simulink model "FluxModel2015a_verify_Q_zhixin"  (R2020b)
settings: Solver=VariableStepAuto  StartTime=0.0  StopTime=0.3  FixedStep=Ts  RelTol=1e-3  EnableMultiTasking=on
model workspace (MAT data in the model file):
  MOVE : Simulink.Parameter (value not decoded)
  STOP : Simulink.Parameter (value not decoded)
  thres : Simulink.Parameter (value not decoded)
values from neighbouring files (symbols this model uses):
  AngleEncoderEn = 1    [parameters.m]
  AngleSpdClosedLoopEnable = 0.0    (= 0)    [parameters.m]
  CurrentLoopMax = Q14*1.2    (= 19660.8)    [parameters.m]
  EstOutMax_Speed_Q = Q14*1.2    (= 19660.8)    [parameters.m]
  Factor1 = Q15*Ts*Rb/Lq_realvalue    [parameters.m]
  Factor2 = Q15*Ts*Rs_realvalue/Lq_realvalue    (= 16990.2962963)    [parameters.m]
  fieldweaken_Max = 0    [parameters.m]
  fieldweaken_Min = -0.5*Q14    (= -8192)    [parameters.m]
  FieldWeakenEn = 0    [parameters.m]
  fluxF = Lam_realvalue/fluxB    [parameters.m]
  fluxF_Q14 = Q14*fluxF    [parameters.m]
  Friction = 0.003    [parameters.m]
  Ib = sqrt(2)*In    [parameters.m]
  Id_Ki = Q14*CurrentLoopBandwidth*Rs    [parameters.m]
  Id_Kp = Q14*CurrentLoopBandwidth*Ld    [parameters.m]
  IFCurrDecreased = 1    [parameters.m]
  IFCurrStart = 8    [parameters.m]
  IFCurrTarget = 5    [parameters.m]
  IFIdref = 0    [parameters.m]
  initial_degree = 0    [parameters.m]
  Iq_Ki = Q14*CurrentLoopBandwidth*Rs    [parameters.m]
  Iq_Kp = Q14*CurrentLoopBandwidth*Lq    [parameters.m]
  J_realvalue = 2.47e-4    (= 0.000247)    [parameters.m]
  KI_fieldweaken = 0.1*Q14    (= 1638.4)    [parameters.m]
  KP_fieldweaken = 1.0*Q14    (= 16384)    [parameters.m]
  LamObserverGain_Q = Q15*LamObserverGain    (= 13106.8)    [parameters.m]
  Ld = Ld_realvalue/Lb    [parameters.m]
  Ld_Q14 = Q14*Ld_realvalue/Lb    [parameters.m]
  Ld_realvalue = 2.7e-3    (= 0.0027)    [parameters.m]
  LowPassFilterBandWidth_Emf_Q = Q14*LowPassFilterBandWidth_Emf    (= 1445.64705882)    [parameters.m]
  LowPassFilterCoeff_Emf = Q15*(1/(1+LowPassFilterBandWidth_Emf*TsPu))    (= 31292.3812732)    [parameters.m]
  LowPassFilterCoeff_Spd = Q15*(1/(1+LowPassFilterBandWidth_Speed*SpeedloopTs/tb))    (= 20123.2126159)    [parameters.m]
  Lq = Lq_realvalue/Lb    [parameters.m]
  Lq_Q14 = Q14*Lq_realvalue/Lb    [parameters.m]
  Lq_realvalue = 2.7e-3    (= 0.0027)    [parameters.m]
  MOVE = 1    [parameters.m]
  Np = 1    [parameters.m]
  Omega0_Q = Q14*Omega0    (= 6553.6)    [parameters.m]
  OverModulationEn = 0    [parameters.m]
  PLL_KI = Q14*PLL_Bandwidth*PLL_Bandwidth    (= 56.6920415225)    [parameters.m]
  PLL_KP = Q14*2*PLL_Bandwidth    (= 1927.52941176)    [parameters.m]
  PLL_OUTMax_W = Q14*1.2    (= 19660.8)    [parameters.m]
  PWM_Period = 1000    [parameters.m]
  Q14 = 16384    [parameters.m]
  Q15 = 32767    [parameters.m]
  Q16 = 65535    [parameters.m]
  Rs = Rs_realvalue/Rb    [parameters.m]
  Rs_Q14 = Q14*Rs_realvalue/Rb    [parameters.m]
  Rs_realvalue = 28    [parameters.m]
  SecondOverMod = 0    [parameters.m]
  SMO_Gain = Q14*0.85    (= 13926.4)    [parameters.m]
  SMO_I_ERROR = Q14*0.05    (= 819.2)    [parameters.m]
  SpdClosedLoopEnable = 0.0    (= 0)    [parameters.m]
  Speed_Ki = Q14*SpeedLoopBandwidth    (= 481.882352941)    [parameters.m]
  Speed_Kp = Q14*SpeedLoopBandwidth*JPu/fluxF    [parameters.m]
  SpeedIncreased = 0.1*Wb    (= 1068.14150222)    [parameters.m]
  SpeedloopTs = 1/SpeedloopFrequency    (= 0.001)    [parameters.m]
  Speedn = 60*fn/Np    (= 102000)    [parameters.m]
  SpeedOutmax = 1.2*Q14    (= 19660.8)    [parameters.m]
  SpeedSwitch = 0.6*Wb    (= 6408.84901332)    [parameters.m]
  SpeedTarget = 0.8*Wb    (= 8545.13201776)    [parameters.m]
  STOP = 0    [parameters.m]
  SVCM_GAIN_Q = Q15*SVCM_GAIN    (= 26213.6)    [parameters.m]
  tb = 1/Wb    (= 9.36205547599e-05)    [parameters.m]
  Tf = 0    [parameters.m]
  thres = 0.1    [parameters.m]
  Tn = 0.012    [parameters.m]
  Ts = 1/SwitchFrequency    (= 5e-05)    [parameters.m]
  TsPu = Ts/tb    (= 0.53407075111)    [parameters.m]
  Vb = Vdc/sqrt(3)    [parameters.m]
  Vdc = sqrt(2)*Un    [parameters.m]
  Wb = 2*pi*fn    (= 10681.4150222)    [parameters.m]
  ZeroSeqInjectEn = 0.0    (= 0)    [parameters.m]
undefined symbols (not defined in the file or in its folder): DiscIntNeverNeededParam, EstOutMax_Theta, magnitude, sigbuilder_block
libraries: simulink x9, powerlib x5, mcbutilslib x1
(part 2 of 3)

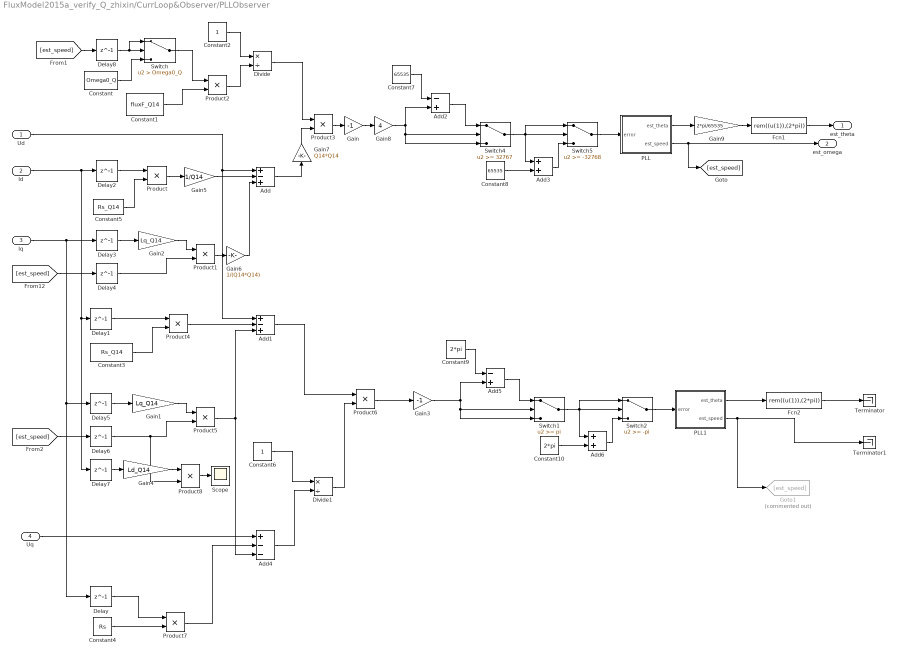
== system FluxModel2015a_verify_Q_zhixin/CurrLoop&Observer/PLLObserver ==
  Ud : Inport
  Id : Inport  Port=2
  Iq : Inport  Port=3
  Uq : Inport  Port=4
  Add : Sum  Inputs=+-+
  Add1 : Sum  Inputs=+-+
  Add2 : Sum  Inputs=-+
  Add3 : Sum
  Add4 : Sum  Inputs=+--
  Add5 : Sum  Inputs=-+
  Add6 : Sum
  Constant : Constant  Value=Omega0_Q
  Constant1 : Constant  Value=fluxF_Q14
  Constant10 : Constant  Value=2*pi
  Constant2 : Constant
  Constant3 : Constant  Value=Rs_Q14
  Constant4 : Constant  Value=Rs
  Constant5 : Constant  Value=Rs_Q14
  Constant6 : Constant
  Constant7 : Constant  Value=65535
  Constant8 : Constant  Value=65535
  Constant9 : Constant  Value=2*pi
  Delay{,1..8} (9 alike) : Delay  DelayLength=1
  Divide : Product  Inputs=*/
  Divide1 : Product  Inputs=*/
  Fcn1 : Fcn  Expr=rem((u(1)),(2*pi))
  Fcn2 : Fcn  Expr=rem((u(1)),(2*pi))
  Gain : Gain  Gain=-1
  Gain1 : Gain  Gain=Lq_Q14
  Gain2 : Gain  Gain=Lq_Q14
  Gain3 : Gain  Gain=-1
  Gain4 : Gain  Gain=Ld_Q14
  Gain5 : Gain  Gain=1/Q14
  Gain6 : Gain  Gain=1/(Q14*Q14)
  Gain7 : Gain  Gain=Q14*Q14
  Gain8 : Gain  Gain=4
  Gain9 : Gain  Gain=2*pi/65535
  Goto1 : Goto  Commented=on  GotoTag=est_speed
  PLL : Subsystem
  PLL1 : Subsystem
  Product{,1..8} (9 alike) : Product
  Scope : Scope
  Switch : Switch  Criteria=u2 > Threshold  Threshold=Omega0_Q
  Switch1 : Switch  Threshold=pi
  Switch2 : Switch  Threshold=-pi
  Switch4 : Switch  Threshold=32767
  Switch5 : Switch  Threshold=-32768
  Terminator : Terminator
  Terminator1 : Terminator
  est_theta : Outport
  est_omega : Outport  Port=2
  wires:
  Constant5/1 -> Product/2
  [est_speed] -> Delay4/1
  Delay4/1 -> Product1/2
  Gain2/1 -> Product1/1
  Delay3/1 -> Gain2/1
  Product1/1 -> Gain6/1
  Product/1 -> Gain5/1
  Delay2/1 -> Product/1
  Id/1 -> Delay7/1, Delay1/1, Delay2/1
  Add/1 -> Gain7/1
  Delay8/1 -> Switch/1, Switch/2
  Constant/1 -> Switch/3
  Switch/1 -> Product2/1
  Constant1/1 -> Product2/2
  Constant2/1 -> Divide/1
  Product2/1 -> Divide/2
  Divide/1 -> Product3/1
  Switch4/1 -> Switch5/1, Add3/1, Switch5/2
  PLL/2(est_speed) -> est_omega/1, [est_speed]
  Add3/1 -> Switch5/3
  Constant8/1 -> Add3/2
  Constant7/1 -> Add2/1
  Add2/1 -> Switch4/1
  Switch5/1 -> PLL/1(error)
  Product3/1 -> Gain/1
  Gain/1 -> Gain8/1
  PLL/1(est_theta) -> Gain9/1
  Constant3/1 -> Product4/2
  Product4/1 -> Add1/2
  Delay1/1 -> Product4/1
  Ud/1 -> Add1/1, Add/1
  Delay6/1 -> Product8/2, Product5/2
  Gain1/1 -> Product5/1
  Delay5/1 -> Gain1/1
  Iq/1 -> Delay/1, Delay5/1, Delay3/1
  Product5/1 -> Add4/3, Add1/3
  Add1/1 -> Product6/1
  Uq/1 -> Add4/1
  Delay/1 -> Product7/1
  Constant4/1 -> Product7/2
  Product7/1 -> Add4/2
  Constant6/1 -> Divide1/1
  Add4/1 -> Divide1/2
  Divide1/1 -> Product6/2
  Product6/1 -> Gain3/1
  Switch1/1 -> Switch2/1, Add6/1, Switch2/2
  Constant9/1 -> Add5/1
  Constant10/1 -> Add6/2
  Switch2/1 -> PLL1/1(error)
  Add5/1 -> Switch1/1
  Gain3/1 -> Switch1/3, Switch1/2, Add5/2
  Add6/1 -> Switch2/3
  PLL1/1(est_theta) -> Fcn2/1
  Fcn2/1 -> Terminator/1
  PLL1/2(est_speed) -> Terminator1/1, Goto1/1
  Fcn1/1 -> est_theta/1
  Delay7/1 -> Gain4/1
  [est_speed] -> Delay6/1
  Gain4/1 -> Product8/1
  Product8/1 -> Scope/1
  Gain5/1 -> Add/2
  Gain6/1 -> Add/3
  Gain7/1 -> Product3/2
  Gain8/1 -> Switch4/3, Switch4/2, Add2/2
  Gain9/1 -> Fcn1/1
  [est_speed] -> Delay8/1

== system FluxModel2015a_verify_Q_zhixin/CurrLoop&Observer/Park ==
  alpha : Inport
  beta : Inport  Port=2
  theta : Inport  Port=3
  Add : Sum
  Cos : Trigonometry  Operator=cos
  Product{,1..3} (4 alike) : Product
  Sin : Trigonometry
  Subtract1 : Sum  Inputs=+-
  ID : Outport
  IQ : Outport  Port=2
  wires:
  Product2/1 -> Subtract1/1
  beta/1 -> Product2/1, Product/1
  theta/1 -> Cos/1, Sin/1
  Sin/1 -> Product3/2, Product/2
  alpha/1 -> Product3/1, Product1/2
  Cos/1 -> Product1/1, Product2/2
  Subtract1/1 -> IQ/1
  Product1/1 -> Add/2
  Product3/1 -> Subtract1/2
  Product/1 -> Add/1
  Add/1 -> ID/1

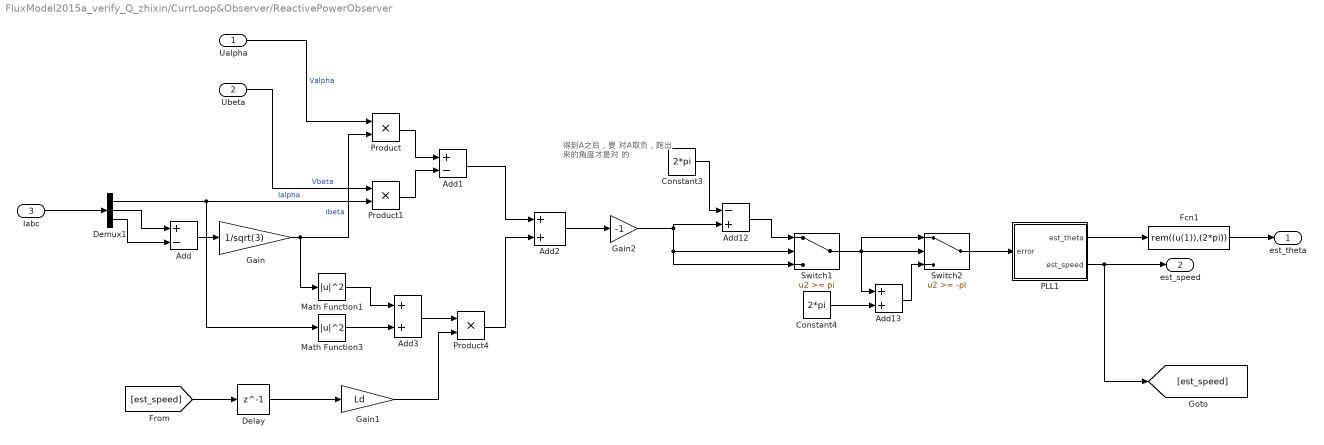
== system FluxModel2015a_verify_Q_zhixin/CurrLoop&Observer/ReactivePowerObserver ==
  note: 得到A之后，要
      | 对A取负，跑出
      | 来的角度才是对
      | 的
  Ualpha : Inport
  Ubeta : Inport  Port=2
  Iabc : Inport  Port=3
  Add : Sum  Inputs=+-
  Add1 : Sum  Inputs=+-
  Add12 : Sum  Inputs=-+
  Add13 : Sum
  Add2 : Sum
  Add3 : Sum
  Constant3 : Constant  Value=2*pi
  Constant4 : Constant  Value=2*pi
  Delay : Delay  DelayLength=1
  Demux1 : Demux  Outputs=3
  Fcn1 : Fcn  Expr=rem((u(1)),(2*pi))
  Gain : Gain  Gain=1/sqrt(3)
  Gain1 : Gain  Gain=Ld
  Gain2 : Gain  Gain=-1
  Math Function1 : Math  Operator=magnitude^2  SaturateOnIntegerOverflow=on
  Math Function3 : Math  Operator=magnitude^2  SaturateOnIntegerOverflow=on
  PLL1 : Subsystem
  Product : Product
  Product1 : Product
  Product4 : Product
  Switch1 : Switch  Threshold=pi
  Switch2 : Switch  Threshold=-pi
  est_theta : Outport
  est_speed : Outport  Port=2
  wires:
  Demux1/1 -> Product1/2, Math Function3/1  "Ialpha"
  Product1/1 -> Add1/2
  Math Function1/1 -> Add3/1
  Demux1/2 -> Add/1
  Gain/1 -> Product/2, Math Function1/1  "Ibeta"
  Add1/1 -> Add2/1
  Ubeta/1 -> Product1/1  "Vbeta"
  Ualpha/1 -> Product/1  "Valpha"
  Product/1 -> Add1/1
  Add/1 -> Gain/1
  Demux1/3 -> Add/2
  Product4/1 -> Add2/2
  Add3/1 -> Product4/1
  Gain1/1 -> Product4/2
  Iabc/1 -> Demux1/1
  Constant4/1 -> Add13/2
  Switch2/1 -> PLL1/1(error)
  Switch1/1 -> Switch2/1, Add13/1, Switch2/2
  PLL1/1(est_theta) -> Fcn1/1
  Constant3/1 -> Add12/1
  Add12/1 -> Switch1/1
  PLL1/2(est_speed) -> [est_speed], est_speed/1
  Add13/1 -> Switch2/3
  Math Function3/1 -> Add3/2
  Fcn1/1 -> est_theta/1
  [est_speed] -> Delay/1
  Delay/1 -> Gain1/1
  Add2/1 -> Gain2/1
  Gain2/1 -> Switch1/3, Switch1/2, Add12/2

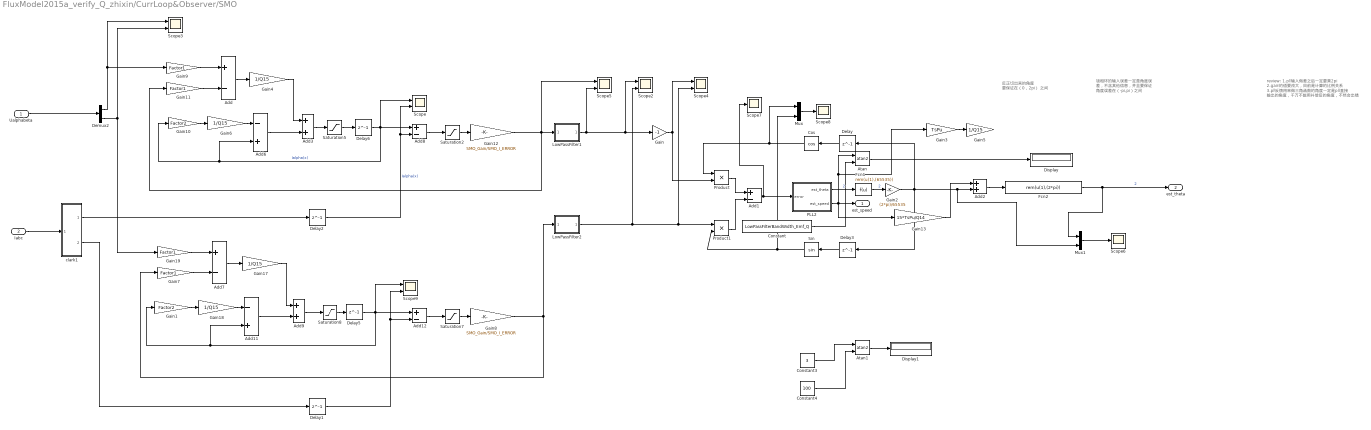
== system FluxModel2015a_verify_Q_zhixin/CurrLoop&Observer/SMO ==
  note: 反正切出来的角度
      | 要保证在（0，2pi）
      | 之间
  note: 锁相环的输入误差一定是角度误
      | 差，不含其他信息，并且要保证
      | 角度误差在（-pi,pi）之间
  note: review:
      | 1.pll输入做差之后一定要乘2pi
      | 2.gain的值要改大，目前是计算的比例关系
      | 3.pll反馈用来做三角函数的角度一定是pll直接
      | 输出的角度，千万不能用补偿后的角度，不然会出错
  Ualphabeta : Inport
  Iabc : Inport  Port=2
  Add{,1,7..8,12} (5 alike) : Sum  Inputs=+-
  Add11 : Sum  Inputs=-+
  Add2 : Sum
  Add3 : Sum
  Add6 : Sum  Inputs=-+
  Add9 : Sum
  Atan : Trigonometry  Operator=atan2
  Atan1 : Trigonometry  Operator=atan2
  Constant : Constant  Value=LowPassFilterBandWidth_Emf_Q
  Constant3 : Constant  Value=3
  Constant4 : Constant  Value=100
  Cos : Trigonometry  Operator=cos
  Delay{,1..3,5..6} (6 alike) : Delay  DelayLength=1
  Demux2 : Demux  Outputs=2
  Display : Display
  Display1 : Display
  Fcn1 : Fcn  Expr=rem(u(1),(65535))
  Fcn2 : Fcn  Expr=rem(u(1),(2*pi))
  Gain : Gain  Gain=-1
  Gain1 : Gain  Gain=Factor2
  Gain10 : Gain  Gain=Factor2
  Gain{7,9,11,19} (4 alike) : Gain  Gain=Factor1
  Gain12 : Gain  Gain=SMO_Gain/SMO_I_ERROR
  Gain13 : Gain  Gain=15*TsPu/Q14
  Gain{4..6,17..18} (5 alike) : Gain  Gain=1/Q15
  Gain2 : Gain  Gain=(2*pi)/65535
  Gain3 : Gain  Gain=TsPu
  Gain8 : Gain  Gain=SMO_Gain/SMO_I_ERROR
  LowPassFilter1 : Subsystem
  LowPassFilter2 : Subsystem
  Mux : Mux  Inputs=2
  Mux1 : Mux  Inputs=2
  PLL2 : Subsystem
  Product : Product
  Product1 : Product
  Saturation2 : Saturate  UpperLimit=SMO_I_ERROR  LowerLimit=-SMO_I_ERROR
  Saturation5 : Saturate  UpperLimit=16384  LowerLimit=-16384
  Saturation7 : Saturate  UpperLimit=SMO_I_ERROR  LowerLimit=-SMO_I_ERROR
  Saturation8 : Saturate  UpperLimit=16384  LowerLimit=-16384
  Scope{,2..5,9} (6 alike) : Scope  NumInputPorts=2
  Scope6 : Scope
  Scope7 : Scope
  Scope8 : Scope
  Sin : Trigonometry
  clark1 : Subsystem
  est_speed : Outport
  est_theta : Outport  Port=2
  wires:
  Demux2/1 -> Scope3/1, Gain9/1
  Gain9/1 -> Add/1
  Saturation2/1 -> Gain12/1
  Gain11/1 -> Add/2
  Add8/1 -> Saturation2/1
  Delay6/1 -> Scope/1, Add8/1, Add6/2, Gain10/1  "Ialpha(x)"
  Delay/1 -> Cos/1
  Cos/1 -> Mux/1, Product/1
  Delay3/1 -> Sin/1
  Sin/1 -> Mux/2, Product1/2
  Product/1 -> Add1/1
  Product1/1 -> Add1/2
  PLL2/2(est_speed) -> Gain13/1, Gain3/1, Atan/1, est_speed/1
  Add1/1 -> PLL2/1(error), Scope7/1
  PLL2/1(est_theta) -> Fcn1/1  "2"
  Constant/1 -> Atan/2
  Fcn2/1 -> Mux1/1, est_theta/1  "2"
  Add2/1 -> Fcn2/1
  Constant3/1 -> Atan1/1
  Constant4/1 -> Atan1/2
  Atan1/1 -> Display1/1
  LowPassFilter1/1(Output) -> Scope5/2, Scope2/1, Gain/1
  Add/1 -> Gain4/1
  Gain4/1 -> Add3/1
  Ualphabeta/1 -> Demux2/1
  Iabc/1 -> clark1/1(Iabc)
  Delay2/1 -> Scope/2, Add8/2  "Ialpha(x)"
  Gain/1 -> Product/2, Scope4/1
  LowPassFilter2/1(Output) -> Scope2/2, Product1/1, Scope4/2
  Mux/1 -> Scope8/1
  Atan/1 -> Display/1
  clark1/1(Ialpha) -> Delay2/1
  Gain12/1 -> Scope5/1, LowPassFilter1/1(Input), Gain11/1
  Add6/1 -> Add3/2
  Gain10/1 -> Gain6/1
  Gain6/1 -> Add6/1
  Add11/1 -> Add9/2
  Gain1/1 -> Gain18/1
  Gain18/1 -> Add11/1
  Gain7/1 -> Add7/2
  clark1/2(Ibeta) -> Delay1/1
  Gain8/1 -> LowPassFilter2/1(Input), Gain7/1
  Saturation7/1 -> Gain8/1
  Add7/1 -> Gain17/1
  Gain17/1 -> Add9/1
  Delay5/1 -> Scope9/1, Add12/1, Add11/2, Gain1/1
  Gain19/1 -> Add7/1
  Demux2/2 -> Gain19/1, Scope3/2
  Add12/1 -> Saturation7/1
  Delay1/1 -> Scope9/2, Add12/2
  Add3/1 -> Saturation5/1
  Saturation5/1 -> Delay6/1
  Add9/1 -> Saturation8/1
  Saturation8/1 -> Delay5/1
  Fcn1/1 -> Gain2/1  "2"
  Mux1/1 -> Scope6/1
  Gain3/1 -> Gain5/1
  Gain2/1 -> Mux1/2, Add2/2, Delay3/1, Delay/1
  Gain13/1 -> Add2/1

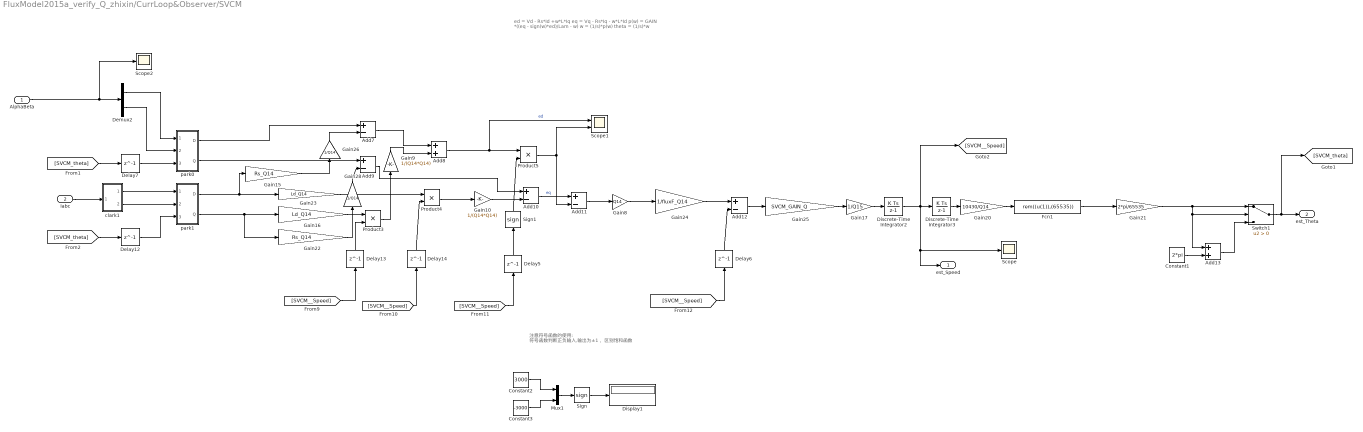
== system FluxModel2015a_verify_Q_zhixin/CurrLoop&Observer/SVCM ==
  note: 注意符号函数的使用:
      | 符号函数判断正负输入,输出为±1，
      | 区别饱和函数
  note: ed = Vd - Rs*Id +w*L*Iq
      | eq = Vq - Rs*Iq - w*L*Id
      | p(w) = GAIN *((eq - sign(w)*ed)/Lam - w)
      | w = (1/s)*p(w)
      | theta = (1/s)*w
  AlphaBeta : Inport
  Iabc : Inport  Port=2
  Add{7,9..12} (5 alike) : Sum  Inputs=+-
  Add13 : Sum
  Add8 : Sum
  Constant1 : Constant  Value=2*pi
  Constant2 : Constant  Value=3000
  Constant3 : Constant  Value=-3000
  Delay{5..7,12..14} (6 alike) : Delay  DelayLength=1
  Demux2 : Demux  Outputs=2
  Discrete-Time Integrator2 : DiscreteIntegrator  gainval=1.0/tb  SampleTime=-1  LimitOutput=on  UpperSaturationLimit=EstOutMax_Speed_Q  LowerSaturationLimit=-EstOutMax_Speed_Q  ICPrevOutput=DiscIntNeverNeededParam  ICPrevScaledInput=DiscIntNeverNeededParam
  Discrete-Time Integrator3 : DiscreteIntegrator  gainval=1.0/tb  SampleTime=-1  UpperSaturationLimit=EstOutMax_Theta  LowerSaturationLimit=-EstOutMax_Theta  ICPrevOutput=DiscIntNeverNeededParam  ICPrevScaledInput=DiscIntNeverNeededParam
  Display1 : Display
      settings: Decimation=2
  Fcn1 : Fcn  Expr=rem((u(1)),(65535))
  Gain10 : Gain  Gain=1/(Q14*Q14)
  Gain15 : Gain  Gain=Rs_Q14
  Gain16 : Gain  Gain=Ld_Q14
  Gain17 : Gain  Gain=1/Q15
  Gain20 : Gain  Gain=10430/Q14
  Gain21 : Gain  Gain=2*pi/65535
  Gain22 : Gain  Gain=Rs_Q14
  Gain23 : Gain  Gain=Ld_Q14
  Gain24 : Gain  Gain=1/fluxF_Q14
  Gain25 : Gain  Gain=SVCM_GAIN_Q
  Gain26 : Gain  Gain=1/Q14
  Gain28 : Gain  Gain=1/Q14
  Gain8 : Gain  Gain=Q14
  Gain9 : Gain  Gain=1/(Q14*Q14)
  Mux1 : Mux  Inputs=2
  Product3 : Product
  Product4 : Product
  Product5 : Product
  Scope : Scope
  Scope1 : Scope  NumInputPorts=2
  Scope2 : Scope
  Sign : Signum
  Sign1 : Signum
  Switch1 : Switch  Criteria=u2 > Threshold
  clark1 : Subsystem
  park0 : Subsystem
  park1 : Subsystem
  est_Speed : Outport
  est_Theta : Outport  Port=2
  wires:
  Gain25/1 -> Gain17/1
  Discrete-Time Integrator3/1 -> Gain20/1
  Product3/1 -> Gain9/1
  Gain26/1 -> Add7/2
  Gain28/1 -> Add9/2
  Switch1/1 -> est_Theta/1, [SVCM_theta]
  Delay14/1 -> Product4/2
  Add13/1 -> Switch1/3
  Demux2/1 -> park0/1(alpha)
  Demux2/2 -> park0/2(beta)
  Delay7/1 -> park0/3(theta)
  Delay12/1 -> park1/3(theta)
  [SVCM_theta] -> Delay7/1
  Gain15/1 -> Gain26/1
  Add11/1 -> Gain8/1
  clark1/2(Ibeta) -> park1/2(beta)
  [SVCM__Speed] -> Delay6/1
  clark1/1(Ialpha) -> park1/1(alpha)
  Product4/1 -> Gain10/1
  Gain22/1 -> Gain28/1
  Add12/1 -> Gain25/1
  Add7/1 -> Add8/1
  Add10/1 -> Add11/1  "eq"
  Add8/1 -> Scope1/1, Product5/1  "ed"
  Constant1/1 -> Add13/2
  [SVCM_theta] -> Delay12/1
  Gain24/1 -> Add12/1
  Gain16/1 -> Product3/1
  Delay6/1 -> Add12/2
  Add9/1 -> Add10/1
  Gain23/1 -> Product4/1
  Delay13/1 -> Product3/2
  Iabc/1 -> clark1/1(Iabc)
  Fcn1/1 -> Gain21/1
  Gain20/1 -> Fcn1/1
  Gain21/1 -> Switch1/1, Add13/1, Switch1/2
  Discrete-Time Integrator2/1 -> Scope/1, est_Speed/1, [SVCM__Speed], Discrete-Time Integrator3/1
  Gain9/1 -> Add8/2
  Gain10/1 -> Add10/2
  [SVCM__Speed] -> Delay13/1
  [SVCM__Speed] -> Delay14/1
  [SVCM__Speed] -> Delay5/1
  Product5/1 -> Add11/2, Scope1/2
  Sign1/1 -> Product5/2
  Delay5/1 -> Sign1/1
  Gain8/1 -> Gain24/1
  Gain17/1 -> Discrete-Time Integrator2/1
  Sign/1 -> Display1/1
  Constant2/1 -> Mux1/1
  Constant3/1 -> Mux1/2
  Mux1/1 -> Sign/1
  AlphaBeta/1 -> Scope2/1, Demux2/1
  park0/1(D) -> Add7/1
  park0/2(Q) -> Add9/1
  park1/1(D) -> Gain23/1, Gain15/1
  park1/2(Q) -> Gain22/1, Gain16/1

== system FluxModel2015a_verify_Q_zhixin/CurrLoop&Observer/Subsystem ==
  err : Inport
  Constant14 : Constant  Value=2*pi
  Constant15 : Constant  Value=pi
  Divide4 : Product  Inputs=*/
  Gain5 : Gain  Gain=180
  Math Function6 : Math  Operator=rem  SaturateOnIntegerOverflow=on
  err_Theta : Outport
  err_Rad : Outport  Port=2
  wires:
  Divide4/1 -> Gain5/1
  Constant15/1 -> Divide4/2
  err/1 -> Math Function6/1
  Math Function6/1 -> err_Rad/1, Divide4/1  "err_Theta"
  Constant14/1 -> Math Function6/2
  Gain5/1 -> err_Theta/1

== system FluxModel2015a_verify_Q_zhixin/CurrLoop&Observer/Subsystem1 ==
  err : Inport
  Constant14 : Constant  Value=2*pi
  Constant15 : Constant  Value=pi
  Divide4 : Product  Inputs=*/
  Gain5 : Gain  Gain=180
  Math Function6 : Math  Operator=rem  SaturateOnIntegerOverflow=on
  err_Theta : Outport
  err_Rad : Outport  Port=2
  wires:
  Gain5/1 -> err_Theta/1
  Constant14/1 -> Math Function6/2
  Math Function6/1 -> Divide4/1, err_Rad/1  "err_Theta"
  err/1 -> Math Function6/1
  Constant15/1 -> Divide4/2
  Divide4/1 -> Gain5/1

== system FluxModel2015a_verify_Q_zhixin/CurrLoop&Observer/Subsystem2 ==
  err : Inport
  Constant14 : Constant  Value=2*pi
  Constant15 : Constant  Value=pi
  Divide4 : Product  Inputs=*/
  Gain5 : Gain  Gain=180
  Math Function6 : Math  Operator=rem  SaturateOnIntegerOverflow=on
  err_Theta : Outport
  err_Rad : Outport  Port=2
  wires:
  Divide4/1 -> Gain5/1
  Constant15/1 -> Divide4/2
  err/1 -> Math Function6/1
  Math Function6/1 -> err_Rad/1, Divide4/1  "err_Theta"
  Constant14/1 -> Math Function6/2
  Gain5/1 -> err_Theta/1

== system FluxModel2015a_verify_Q_zhixin/CurrLoop&Observer/Subsystem3 ==
  err : Inport
  Constant14 : Constant  Value=2*pi
  Constant15 : Constant  Value=pi
  Divide4 : Product  Inputs=*/
  Gain5 : Gain  Gain=180
  Math Function6 : Math  Operator=rem  SaturateOnIntegerOverflow=on
  err_Theta : Outport
  err_Rad : Outport  Port=2
  wires:
  Gain5/1 -> err_Theta/1
  Constant14/1 -> Math Function6/2
  Math Function6/1 -> Divide4/1, err_Rad/1  "err_Theta"
  err/1 -> Math Function6/1
  Constant15/1 -> Divide4/2
  Divide4/1 -> Gain5/1

== system FluxModel2015a_verify_Q_zhixin/CurrLoop&Observer/Subsystem4 ==
  err : Inport
  Constant14 : Constant  Value=2*pi
  Constant15 : Constant  Value=pi
  Divide4 : Product  Inputs=*/
  Gain5 : Gain  Gain=180
  Math Function6 : Math  Operator=rem  SaturateOnIntegerOverflow=on
  err_Theta : Outport
  err_Rad : Outport  Port=2
  wires:
  Divide4/1 -> Gain5/1
  Constant15/1 -> Divide4/2
  err/1 -> Math Function6/1
  Math Function6/1 -> err_Rad/1, Divide4/1  "err_Theta"
  Constant14/1 -> Math Function6/2
  Gain5/1 -> err_Theta/1

== system FluxModel2015a_verify_Q_zhixin/CurrLoop&Observer/Subsystem5 ==
  err : Inport
  Gain1 : Gain  Gain=Wb
  Gain2 : Gain  Gain=1/(2*pi)
  Gain3 : Gain  Gain=60/Np
  err_Spd : Outport
  err_Fhz : Outport  Port=2
  wires:
  err/1 -> Gain1/1
  Gain2/1 -> err_Fhz/1, Gain3/1
  Gain1/1 -> Gain2/1
  Gain3/1 -> err_Spd/1

== system FluxModel2015a_verify_Q_zhixin/CurrLoop&Observer/Subsystem6 ==
  err : Inport
  Gain1 : Gain  Gain=Wb
  Gain2 : Gain  Gain=1/(2*pi)
  Gain3 : Gain  Gain=60/Np
  err_Spd : Outport
  err_Fhz : Outport  Port=2
  wires:
  Gain3/1 -> err_Spd/1
  Gain1/1 -> Gain2/1
  Gain2/1 -> Gain3/1, err_Fhz/1
  err/1 -> Gain1/1

== system FluxModel2015a_verify_Q_zhixin/CurrLoop&Observer/Subsystem7 ==
  err : Inport
  Gain1 : Gain  Gain=Wb
  Gain2 : Gain  Gain=1/(2*pi)
  Gain3 : Gain  Gain=60/Np
  err_Spd : Outport
  err_Fhz : Outport  Port=2
  wires:
  err/1 -> Gain1/1
  Gain2/1 -> err_Fhz/1, Gain3/1
  Gain1/1 -> Gain2/1
  Gain3/1 -> err_Spd/1

== system FluxModel2015a_verify_Q_zhixin/CurrLoop&Observer/Subsystem8 ==
  err : Inport
  Gain1 : Gain  Gain=Wb
  Gain2 : Gain  Gain=1/(2*pi)
  Gain3 : Gain  Gain=60/Np
  err_Spd : Outport
  err_Fhz : Outport  Port=2
  wires:
  Gain3/1 -> err_Spd/1
  Gain1/1 -> Gain2/1
  Gain2/1 -> Gain3/1, err_Fhz/1
  err/1 -> Gain1/1

== system FluxModel2015a_verify_Q_zhixin/CurrLoop&Observer/Subsystem9 ==
  err : Inport
  Gain1 : Gain  Gain=Wb
  Gain2 : Gain  Gain=1/(2*pi)
  Gain3 : Gain  Gain=60/Np
  err_Spd : Outport
  err_Fhz : Outport  Port=2
  wires:
  err/1 -> Gain1/1
  Gain2/1 -> err_Fhz/1, Gain3/1
  Gain1/1 -> Gain2/1
  Gain3/1 -> err_Spd/1

== system FluxModel2015a_verify_Q_zhixin/CurrLoop&Observer/ai-park ==
  UD : Inport
  UQ : Inport  Port=2
  The : Inport  Port=3
  Add : Sum
  Cos : Trigonometry  Operator=cos
  Product{,1..3} (4 alike) : Product
  Sin : Trigonometry
  Subtract : Sum  Inputs=+-
  Valpha : Outport
  Vbeta : Outport  Port=2
  wires:
  UQ/1 -> Product3/1, Product1/1
  Product1/1 -> Subtract/2
  Product3/1 -> Add/2
  Cos/1 -> Product3/2, Product/2
  Sin/1 -> Product2/2, Product1/2
  Product/1 -> Subtract/1
  Product2/1 -> Add/1
  The/1 -> Sin/1, Cos/1
  UD/1 -> Product/1, Product2/1
  Subtract/1 -> Valpha/1
  Add/1 -> Vbeta/1

== system FluxModel2015a_verify_Q_zhixin/CurrLoop&Observer/clark ==
  Iabc : Inport
  Add : Sum  Inputs=+-
  Demux2 : Demux  Outputs=3
  Gain : Gain  Gain=18919
  Gain1 : Gain  Gain=1/Q15
  Ialpha : Outport
  Ibeta : Outport  Port=2
  wires:
  Demux2/3 -> Add/2
  Add/1 -> Gain/1
  Demux2/1 -> Ialpha/1
  Demux2/2 -> Add/1
  Gain/1 -> Gain1/1
  Iabc/1 -> Demux2/1
  Gain1/1 -> Ibeta/1

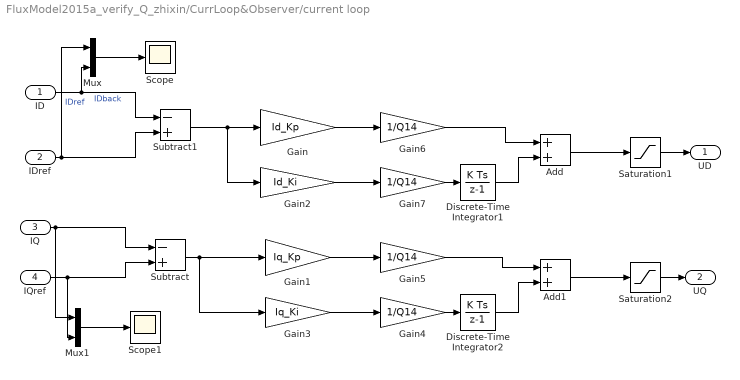
== system FluxModel2015a_verify_Q_zhixin/CurrLoop&Observer/current loop ==
  ID : Inport
  IDref : Inport  Port=2
  IQ : Inport  Port=3
  IQref : Inport  Port=4
  Add : Sum
  Add1 : Sum
  Discrete-Time Integrator1 : DiscreteIntegrator  gainval=1/tb  SampleTime=-1  LimitOutput=on  UpperSaturationLimit=CurrentLoopMax  LowerSaturationLimit=-CurrentLoopMax  ICPrevOutput=DiscIntNeverNeededParam  ICPrevScaledInput=DiscIntNeverNeededParam
  Discrete-Time Integrator2 : DiscreteIntegrator  gainval=1/tb  SampleTime=-1  LimitOutput=on  UpperSaturationLimit=CurrentLoopMax  LowerSaturationLimit=-CurrentLoopMax  ICPrevOutput=DiscIntNeverNeededParam  ICPrevScaledInput=DiscIntNeverNeededParam
  Gain : Gain  Gain=Id_Kp
  Gain1 : Gain  Gain=Iq_Kp
  Gain2 : Gain  Gain=Id_Ki
  Gain3 : Gain  Gain=Iq_Ki
  Gain{4..7} (4 alike) : Gain  Gain=1/Q14
  Mux : Mux  Inputs=2
  Mux1 : Mux  Inputs=2
  Saturation1 : Saturate  UpperLimit=CurrentLoopMax  LowerLimit=-CurrentLoopMax
  Saturation2 : Saturate  UpperLimit=CurrentLoopMax  LowerLimit=-CurrentLoopMax
  Scope : Scope
  Scope1 : Scope
  Subtract : Sum  Inputs=-+
  Subtract1 : Sum  Inputs=-+
  UD : Outport
  UQ : Outport  Port=2
  wires:
  Saturation1/1 -> UD/1
  Subtract1/1 -> Gain/1, Gain2/1
  Saturation2/1 -> UQ/1
  Gain1/1 -> Gain5/1
  Subtract/1 -> Gain3/1, Gain1/1
  Gain/1 -> Gain6/1
  Discrete-Time Integrator1/1 -> Add/2
  Discrete-Time Integrator2/1 -> Add1/2
  IQref/1 -> Mux1/2, Subtract/2
  IDref/1 -> Mux/1, Subtract1/2  "IDref"
  ID/1 -> Mux/2, Subtract1/1  "IDback"
  Mux/1 -> Scope/1
  IQ/1 -> Mux1/1, Subtract/1
  Mux1/1 -> Scope1/1
  Gain3/1 -> Gain4/1
  Add/1 -> Saturation1/1
  Add1/1 -> Saturation2/1
  Gain5/1 -> Add1/1
  Gain4/1 -> Discrete-Time Integrator2/1
  Gain6/1 -> Add/1
  Gain2/1 -> Gain7/1
  Gain7/1 -> Discrete-Time Integrator1/1

== system FluxModel2015a_verify_Q_zhixin/SVPWM/Subsystem ==
  Valpha : Inport
  Vbeta : Inport  Port=2
  Add : Sum  Inputs=+-
  Add1 : Sum  Inputs=+-
  Add2 : Sum  Inputs=+++
  Constant : Constant
  Constant1 : Constant  Value=0
  Gain : Gain  Gain=sqrt(3)
  Gain1 : Gain  Gain=-1
  Gain2 : Gain  Gain=2
  Gain3 : Gain  Gain=4
  Saturation : Saturate  UpperLimit=6  LowerLimit=1
  Switch : Switch  Criteria=u2 > Threshold
  Switch1 : Switch  Criteria=u2 > Threshold
  Switch2 : Switch  Criteria=u2 > Threshold
  N : Outport
  wires:
  Add2/1 -> Saturation/1
  Valpha/1 -> Gain/1
  Gain3/1 -> Add2/2
  Gain2/1 -> Add2/1
  Add1/1 -> Switch1/2
  Gain1/1 -> Add1/1
  Switch1/1 -> Gain3/1
  Switch2/1 -> Add2/3
  Switch/1 -> Gain2/1
  Add/1 -> Switch/2
  Gain/1 -> Gain1/1, Add/1
  Constant1/1 -> Switch/3, Switch1/3, Switch2/3
  Constant/1 -> Switch1/1, Switch2/1, Switch/1
  Vbeta/1 -> Add1/2, Add/2, Switch2/2
  Saturation/1 -> N/1

== system FluxModel2015a_verify_Q_zhixin/SVPWM/Subsystem1 ==
  T : Inport
  In2 : Inport  Port=2
  In3 : Inport  Port=3
  Vdc : Inport  Port=4
  Add : Sum
  Add1 : Sum  Inputs=+-
  Divide : Product  Inputs=**/
  Divide1 : Product  Inputs=**/
  Divide2 : Product  Inputs=**/
  Gain : Gain  Gain=1.732
  Gain1 : Gain  Gain=1.5
  Gain2 : Gain  Gain=0.5
  x : Outport
  Y : Outport  Port=2
  Z : Outport  Port=3
  wires:
  Divide2/1 -> Z/1
  Divide1/1 -> Y/1
  Divide/1 -> x/1
  In3/1 -> Gain1/1
  In2/1 -> Gain/1
  Add1/1 -> Divide2/2
  Add/1 -> Divide1/2
  Gain1/1 -> Add1/2, Add/2
  Gain2/1 -> Add1/1, Add/1
  Gain/1 -> Gain2/1, Divide/2
  Vdc/1 -> Divide/3, Divide1/3, Divide2/3
  T/1 -> Divide2/1, Divide1/1, Divide/1

== system FluxModel2015a_verify_Q_zhixin/SVPWM/Subsystem2 ==
  In1 : Inport
  In2 : Inport  Port=2
  In3 : Inport  Port=3
  In4 : Inport  Port=4
  Gain : Gain  Gain=-1
  Gain1 : Gain  Gain=-1
  Gain2 : Gain  Gain=-1
  Multiport Switch : MultiPortSwitch  Inputs=6
  Multiport Switch1 : MultiPortSwitch  Inputs=6
  T1 : Outport
  T2 : Outport  Port=2
  wires:
  Gain2/1 -> Multiport Switch/7, Multiport Switch1/6
  Gain1/1 -> Multiport Switch1/3, Multiport Switch/5
  In2/1 -> Gain1/1, Multiport Switch/6, Multiport Switch1/4
  Gain/1 -> Multiport Switch1/7, Multiport Switch/4
  In3/1 -> Gain2/1, Multiport Switch1/2, Multiport Switch/3
  In4/1 -> Gain/1, Multiport Switch/2, Multiport Switch1/5
  In1/1 -> Multiport Switch/1, Multiport Switch1/1
  Multiport Switch/1 -> T1/1
  Multiport Switch1/1 -> T2/1

== system FluxModel2015a_verify_Q_zhixin/SVPWM/Subsystem3 ==
  T1 : Inport
  T : Inport  Port=2
  T2 : Inport  Port=3
  Add : Sum  Inputs=--+
  Add1 : Sum
  Add2 : Sum
  Gain : Gain  Gain=0.25
  Gain1 : Gain  Gain=0.5
  Gain2 : Gain  Gain=0.5
  Saturation : Saturate  UpperLimit=Ts/2  LowerLimit=0
  Saturation1 : Saturate  UpperLimit=Ts/2  LowerLimit=0
  Saturation2 : Saturate  UpperLimit=Ts/2  LowerLimit=0
  Ta : Outport
  Tb : Outport  Port=2
  Tc : Outport  Port=3
  wires:
  T/1 -> Add/3
  Gain2/1 -> Add2/2
  Gain1/1 -> Add1/2
  Add/1 -> Gain/1
  T2/1 -> Add/2, Gain2/1
  T1/1 -> Add/1, Gain1/1
  Gain/1 -> Saturation/1, Add1/1
  Add1/1 -> Saturation1/1, Add2/1
  Add2/1 -> Saturation2/1
  Saturation/1 -> Ta/1
  Saturation1/1 -> Tb/1
  Saturation2/1 -> Tc/1

== system FluxModel2015a_verify_Q_zhixin/SVPWM/Subsystem4 ==
  In1 : Inport
  In2 : Inport  Port=2
  In3 : Inport  Port=3
  In4 : Inport  Port=4
  Multiport Switch : MultiPortSwitch  Inputs=6
  Multiport Switch1 : MultiPortSwitch  Inputs=6
  Multiport Switch2 : MultiPortSwitch  Inputs=6
  Saturation : Saturate  UpperLimit=Ts/2  LowerLimit=0
  Saturation1 : Saturate  UpperLimit=Ts/2  LowerLimit=0
  Saturation3 : Saturate  UpperLimit=Ts/2  LowerLimit=0
  Tcm1 : Outport
  Tcm2 : Outport  Port=2
  Tcm3 : Outport  Port=3
  wires:
  In1/1 -> Multiport Switch2/1, Multiport Switch1/1, Multiport Switch/1
  In4/1 -> Multiport Switch1/3, Multiport Switch1/7, Multiport Switch2/2, Multiport Switch2/4, Multiport Switch/5, Multiport Switch/6
  In2/1 -> Multiport Switch/4, Multiport Switch/3, Multiport Switch1/2, Multiport Switch1/6, Multiport Switch2/5, Multiport Switch2/7
  In3/1 -> Multiport Switch/2, Multiport Switch/7, Multiport Switch1/4, Multiport Switch1/5, Multiport Switch2/3, Multiport Switch2/6
  Multiport Switch2/1 -> Saturation3/1
  Saturation3/1 -> Tcm3/1
  Multiport Switch1/1 -> Saturation1/1
  Saturation1/1 -> Tcm2/1
  Multiport Switch/1 -> Saturation/1
  Saturation/1 -> Tcm1/1

== system FluxModel2015a_verify_Q_zhixin/SVPWM/Subsystem5 ==
  In1 : Inport
  In2 : Inport  Port=2
  In3 : Inport  Port=3
  In4 : Inport  Port=4
  Add : Sum  Inputs=+-
  Add1 : Sum  Inputs=+-
  Add2 : Sum  Inputs=+-
  Data Type Conversion : DataTypeConversion  OutDataTypeStr=double
  Data Type Conversion1 : DataTypeConversion  OutDataTypeStr=double
  Data Type Conversion2 : DataTypeConversion  OutDataTypeStr=double
  Logical Operator : Logic  Operator=NOT  AllPortsSameDT=off  OutDataTypeStr=boolean
  Logical Operator1 : Logic  Operator=NOT  AllPortsSameDT=off  OutDataTypeStr=boolean
  Logical Operator2 : Logic  Operator=NOT  AllPortsSameDT=off  OutDataTypeStr=boolean
  Mux : Mux  Inputs=6
  Relay : Relay  OffSwitchValue=-eps
  Relay1 : Relay  OffSwitchValue=-eps
  Relay2 : Relay  OffSwitchValue=-eps
  Unit Delay : UnitDelay  SampleTime=-1  HasFrameUpgradeWarning=on
  Unit Delay1 : UnitDelay  SampleTime=-1  HasFrameUpgradeWarning=on
  Unit Delay2 : UnitDelay  SampleTime=-1  HasFrameUpgradeWarning=on
  g : Outport
  wires:
  In4/1 -> Add2/2
  In3/1 -> Add1/2
  In2/1 -> Add/2
  Relay2/1 -> Unit Delay2/1
  Relay1/1 -> Unit Delay1/1
  Relay/1 -> Unit Delay/1
  Unit Delay2/1 -> Mux/5, Logical Operator2/1
  Unit Delay1/1 -> Mux/3, Logical Operator1/1
  Unit Delay/1 -> Logical Operator/1, Mux/1
  Mux/1 -> g/1
  Data Type Conversion/1 -> Mux/2
  Data Type Conversion1/1 -> Mux/4
  Data Type Conversion2/1 -> Mux/6
  Logical Operator2/1 -> Data Type Conversion2/1
  Logical Operator1/1 -> Data Type Conversion1/1
  Logical Operator/1 -> Data Type Conversion/1
  Add1/1 -> Relay1/1
  Add2/1 -> Relay2/1
  Add/1 -> Relay/1
  In1/1 -> Add/1, Add2/1, Add1/1

== system FluxModel2015a_verify_Q_zhixin/SVPWM/Subsystem6 ==
  T1 : Inport
  T : Inport  Port=2
  T2 : Inport  Port=3
  Add : Sum  Inputs=--+
  Add1 : Sum
  Add2 : Sum
  Gain : Gain  Gain=0.25
  Gain1 : Gain  Gain=0.5
  Gain2 : Gain  Gain=0.5
  Saturation : Saturate  UpperLimit=Ts/2  LowerLimit=0
  Saturation1 : Saturate  UpperLimit=Ts/2  LowerLimit=0
  Saturation2 : Saturate  UpperLimit=Ts/2  LowerLimit=0
  Ta : Outport
  Tb : Outport  Port=2
  Tc : Outport  Port=3
  wires:
  T/1 -> Add/3
  Gain2/1 -> Add2/2
  Gain1/1 -> Add1/2
  Add/1 -> Gain/1
  T2/1 -> Add/2, Gain2/1
  T1/1 -> Add/1, Gain1/1
  Gain/1 -> Saturation/1, Add1/1
  Add1/1 -> Saturation1/1, Add2/1
  Add2/1 -> Saturation2/1
  Saturation/1 -> Ta/1
  Saturation1/1 -> Tb/1
  Saturation2/1 -> Tc/1

== system FluxModel2015a_verify_Q_zhixin/SVPWM/VoltReconstruct ==
  CCR1 : Inport
  CCR2 : Inport  Port=2
  CCR3 : Inport  Port=3
  Add : Sum  Inputs=+--
  Add1 : Sum  Inputs=+--
  Add2 : Sum  Inputs=+--
  Gain : Gain  Gain=1/3
  Gain2 : Gain  Gain=2
  Gain4 : Gain  Gain=2
  Gain5 : Gain  Gain=2
  Mux : Mux  Inputs=3
  Mux1 : Mux  Inputs=3
  Subsystem6 : Subsystem
  Subsystem7 : Subsystem
  Subsystem8 : Subsystem
  Uanbncn : Outport
  Uaoboco : Outport  Port=2
  wires:
  Subsystem7/1(Ubo) -> Mux1/2, Add2/3, Gain4/1, Add/2
  CCR3/1 -> Subsystem8/1(CCR3)
  CCR2/1 -> Subsystem7/1(CCR2)
  Gain4/1 -> Add1/1
  Subsystem8/1(Uco) -> Mux1/3, Add/3, Add1/3, Gain5/1
  Subsystem6/1(Uao) -> Mux1/1, Gain2/1, Add2/2, Add1/2
  CCR1/1 -> Subsystem6/1(CCR1)
  Gain2/1 -> Add/1
  Gain5/1 -> Add2/1
  Add/1 -> Mux/1  "A"
  Add1/1 -> Mux/2  "B"
  Add2/1 -> Mux/3  "C"
  Mux/1 -> Gain/1
  Gain/1 -> Uanbncn/1
  Mux1/1 -> Uaoboco/1

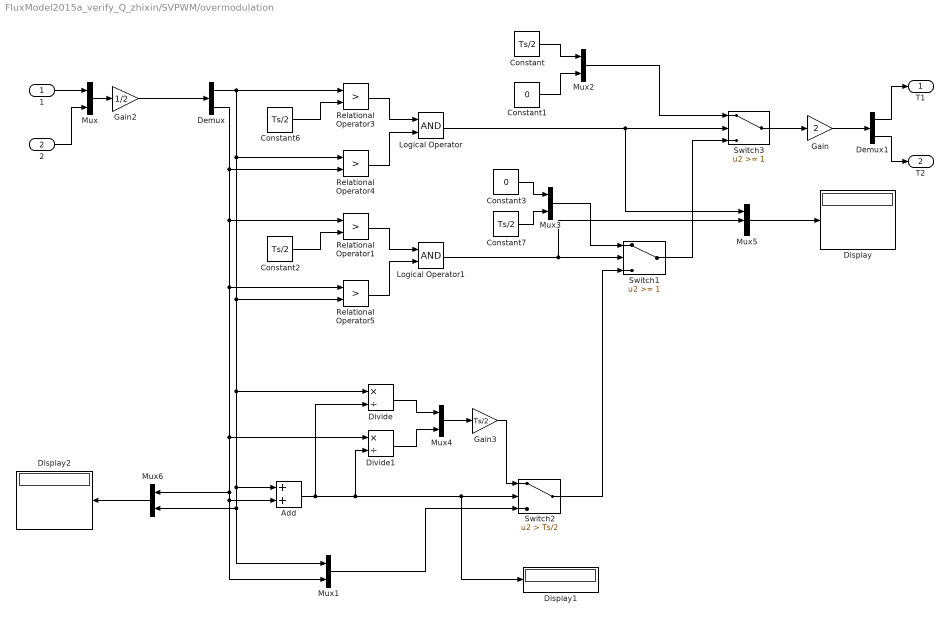
== system FluxModel2015a_verify_Q_zhixin/SVPWM/overmodulation ==
  1 : Inport
  2 : Inport  Port=2
  Add : Sum
  Constant{,2,6..7} (4 alike) : Constant  Value=Ts/2
  Constant1 : Constant  Value=0
  Constant3 : Constant  Value=0
  Demux : Demux  Outputs=2
  Demux1 : Demux  Outputs=2
  Display : Display
  Display1 : Display
  Display2 : Display
  Divide : Product  Inputs=*/
  Divide1 : Product  Inputs=*/
  Gain : Gain  Gain=2
  Gain2 : Gain  Gain=1/2
  Gain3 : Gain  Gain=Ts/2
  Logical Operator : Logic  AllPortsSameDT=off  OutDataTypeStr=boolean
  Logical Operator1 : Logic  AllPortsSameDT=off  OutDataTypeStr=boolean
  Mux{,1..4,6} (6 alike) : Mux  Inputs=2
  Mux5 : Mux  Inputs=3
  Relational Operator{1,3..5} (4 alike) : RelationalOperator  Operator=>  OutDataTypeStr=boolean  RndMeth=Simplest
  Switch1 : Switch  Threshold=1
  Switch2 : Switch  Criteria=u2 > Threshold  Threshold=Ts/2
  Switch3 : Switch  Threshold=1
  T1 : Outport
  T2 : Outport  Port=2
  wires:
  Switch1/1 -> Switch3/3
  Constant3/1 -> Mux3/1
  Divide/1 -> Mux4/1
  Mux/1 -> Gain2/1
  Logical Operator1/1 -> Mux5/2, Switch1/2
  Switch2/1 -> Switch1/3
  Add/1 -> Divide/2, Divide1/2, Display1/1, Switch2/2
  Demux/1 -> Relational Operator4/1, Relational Operator5/2, Divide/1, Mux1/1, Mux6/2, Add/1, Relational Operator3/1
  Mux4/1 -> Gain3/1
  Divide1/1 -> Mux4/2
  Relational Operator1/1 -> Logical Operator1/1
  Constant7/1 -> Mux3/2
  Demux/2 -> Relational Operator4/2, Relational Operator1/1, Relational Operator5/1, Divide1/1, Mux6/1, Mux1/2, Add/2
  Mux2/1 -> Switch3/1
  Gain2/1 -> Demux/1
  Relational Operator3/1 -> Logical Operator/1
  Relational Operator4/1 -> Logical Operator/2
  Relational Operator5/1 -> Logical Operator1/2
  Constant/1 -> Mux2/1
  Constant6/1 -> Relational Operator3/2
  Gain3/1 -> Switch2/1
  Constant2/1 -> Relational Operator1/2
  Constant1/1 -> Mux2/2
  Logical Operator/1 -> Mux5/1, Switch3/2
  Mux3/1 -> Switch1/1
  1/1 -> Mux/1
  2/1 -> Mux/2
  Demux1/1 -> T1/1
  Demux1/2 -> T2/1
  Mux1/1 -> Switch2/3
  Mux5/1 -> Display/1
  Switch3/1 -> Gain/1
  Gain/1 -> Demux1/1
  Mux6/1 -> Display2/1

== system FluxModel2015a_verify_Q_zhixin/SpeedLoop/FieldWeaken ==
  UDUQ : Inport
  Add4 : Sum
  Add5 : Sum  Inputs=+-
  Add6 : Sum
  Constant : Constant  Value=Vdc/sqrt(3)/Vb
  Delay : Delay  DelayLength=1
  Demux : Demux  Outputs=2
  Discrete-Time Integrator : DiscreteIntegrator  gainval=1.0/tb  SampleTime=-1  LimitOutput=on  UpperSaturationLimit=fieldweaken_Max  LowerSaturationLimit=fieldweaken_Min  ICPrevOutput=DiscIntNeverNeededParam  ICPrevScaledInput=DiscIntNeverNeededParam
  Gain : Gain  Gain=KP_fieldweaken
  Gain1 : Gain  Gain=Q14
  Gain2 : Gain  Gain=KI_fieldweaken
  Gain3 : Gain  Gain=1/Q14
  Gain4 : Gain  Gain=1/Q14
  Saturation : Saturate  UpperLimit=fieldweaken_Max  LowerLimit=fieldweaken_Min
  Sqrt1 : Sqrt  SaturateOnIntegerOverflow=on
  Square1 : Math  Operator=square  SaturateOnIntegerOverflow=on
  ID : Outport
  wires:
  Delay/1 -> Square1/1
  Demux/2 -> Add4/2
  Add5/1 -> Gain2/1, Gain/1
  Add4/1 -> Sqrt1/1
  Square1/1 -> Demux/1
  Add6/1 -> Saturation/1
  Discrete-Time Integrator/1 -> Add6/2
  UDUQ/1 -> Delay/1
  Saturation/1 -> ID/1
  Demux/1 -> Add4/1
  Constant/1 -> Gain1/1
  Gain/1 -> Gain3/1
  Gain2/1 -> Gain4/1
  Sqrt1/1 -> Add5/2
  Gain3/1 -> Add6/1
  Gain4/1 -> Discrete-Time Integrator/1
  Gain1/1 -> Add5/1

== system FluxModel2015a_verify_Q_zhixin/SpeedLoop/LowPassFilter2 ==
  Input : Inport
  Add : Sum  Inputs=+-
  Add1 : Sum
  Constant : Constant  Value=32767
  Constant1 : Constant  Value=LowPassFilterCoeff_Spd
  Delay6 : Delay  DelayLength=1
  Gain : Gain  Gain=LowPassFilterCoeff_Spd
  Gain3 : Gain  Gain=1/Q15
  Product : Product
  Output : Outport
  wires:
  Add1/1 -> Gain3/1
  Gain/1 -> Add1/2
  Product/1 -> Add1/1
  Add/1 -> Product/2
  Input/1 -> Product/1
  Constant1/1 -> Add/2
  Constant/1 -> Add/1
  Delay6/1 -> Gain/1
  Gain3/1 -> Output/1, Delay6/1

== system FluxModel2015a_verify_Q_zhixin/SpeedLoop/MTPA ==
  IQ : Inport
  Add4 : Sum
  Add5 : Sum  Inputs=+-
  Constant : Constant  Value=(fluxF^2)/(4*((Ld-Lq)^2))
  Constant1 : Constant  Value=fluxF/(2*(Lq-Ld))
  Sqrt1 : Sqrt  SaturateOnIntegerOverflow=on
  Square : Math  Operator=square  SaturateOnIntegerOverflow=on
  ID : Outport
  wires:
  Sqrt1/1 -> Add5/2
  Square/1 -> Add4/1
  Add4/1 -> Sqrt1/1
  Constant1/1 -> Add5/1
  Constant/1 -> Add4/2
  Add5/1 -> ID/1
  IQ/1 -> Square/1

== system FluxModel2015a_verify_Q_zhixin/SpeedLoop/OpenLoop ==
  CurrDecreased : Inport
  CurrTarget : Inport  Port=2
  CurrStart : Inport  Port=3
  SpdIncreased : Inport  Port=4
  SpdTarget : Inport  Port=5
  Add : Sum
  Add1 : Sum  Inputs=+-
  Constant : Constant  Value=IFIdref
  Delay : Delay  DelayLength=1
  Delay1 : Delay  DelayLength=1  InitialCondition=IFCurrStart
  Gain : Gain  Gain=1/Wb
  Gain1 : Gain  Gain=1/Ib
  Gain8 : Gain  Gain=1/Ib
  Scope : Scope
  Switch2 : Switch  Criteria=u2 > Threshold  Threshold=SpeedSwitch
  Switch3 : Switch  Criteria=u2 > Threshold  Threshold=IFCurrTarget
  Switch4 : Switch  Criteria=u2 > Threshold  Threshold=SpeedTarget
  OpenLoopIQ : Outport
  OpenLoopID : Outport  Port=2
  OpenLoopSpeed : Outport  Port=3
  wires:
  Delay1/1 -> Switch3/1, Switch3/2, Add1/1
  CurrDecreased/1 -> Add1/2
  Add1/1 -> Delay1/1
  SpdTarget/1 -> Switch4/1
  Delay/1 -> Switch4/3, Switch4/2, Switch2/2, Add/1
  Switch3/1 -> Scope/1, Switch2/1
  SpdIncreased/1 -> Add/2
  Add/1 -> Delay/1
  CurrStart/1 -> Switch2/3
  Switch2/1 -> Gain8/1
  Gain8/1 -> OpenLoopIQ/1
  Switch4/1 -> Gain/1
  Gain/1 -> OpenLoopSpeed/1
  CurrTarget/1 -> Switch3/3
  Constant/1 -> Gain1/1
  Gain1/1 -> OpenLoopID/1

== system FluxModel2015a_verify_Q_zhixin/Zero-sequence injection/Subsystem5 ==
  In1 : Inport
  In2 : Inport  Port=2
  In3 : Inport  Port=3
  In4 : Inport  Port=4
  Add : Sum  Inputs=+-
  Add1 : Sum  Inputs=+-
  Add2 : Sum  Inputs=+-
  Data Type Conversion : DataTypeConversion  OutDataTypeStr=double
  Data Type Conversion1 : DataTypeConversion  OutDataTypeStr=double
  Data Type Conversion2 : DataTypeConversion  OutDataTypeStr=double
  Logical Operator : Logic  Operator=NOT  AllPortsSameDT=off  OutDataTypeStr=boolean
  Logical Operator1 : Logic  Operator=NOT  AllPortsSameDT=off  OutDataTypeStr=boolean
  Logical Operator2 : Logic  Operator=NOT  AllPortsSameDT=off  OutDataTypeStr=boolean
  Mux : Mux  Inputs=6
  Relay : Relay  OffSwitchValue=-eps
  Relay1 : Relay  OffSwitchValue=-eps
  Relay2 : Relay  OffSwitchValue=-eps
  Unit Delay : UnitDelay  SampleTime=-1  HasFrameUpgradeWarning=on
  Unit Delay1 : UnitDelay  SampleTime=-1  HasFrameUpgradeWarning=on
  Unit Delay2 : UnitDelay  SampleTime=-1  HasFrameUpgradeWarning=on
  g : Outport
  wires:
  In4/1 -> Add2/2
  In3/1 -> Add1/2
  In2/1 -> Add/2
  Relay2/1 -> Unit Delay2/1
  Relay1/1 -> Unit Delay1/1
  Relay/1 -> Unit Delay/1
  Unit Delay2/1 -> Mux/5, Logical Operator2/1
  Unit Delay1/1 -> Mux/3, Logical Operator1/1
  Unit Delay/1 -> Logical Operator/1, Mux/1
  Mux/1 -> g/1
  Data Type Conversion/1 -> Mux/2
  Data Type Conversion1/1 -> Mux/4
  Data Type Conversion2/1 -> Mux/6
  Logical Operator2/1 -> Data Type Conversion2/1
  Logical Operator1/1 -> Data Type Conversion1/1
  Logical Operator/1 -> Data Type Conversion/1
  Add1/1 -> Relay1/1
  Add2/1 -> Relay2/1
  Add/1 -> Relay/1
  In1/1 -> Add/1, Add2/1, Add1/1

== system FluxModel2015a_verify_Q_zhixin/Zero-sequence injection/antiClarke ==
  Ualpha : Inport
  Ubeta : Inport  Port=2
  Add4 : Sum  Inputs=+-
  Add5 : Sum
  Gain15 : Gain  Gain=(sqrt(3))/2
  Gain16 : Gain  Gain=1/2
  Gain17 : Gain  Gain=-(sqrt(3))/2
  Gain18 : Gain  Gain=-1/2
  Mux4 : Mux  Inputs=3
  Uabc : Outport
  wires:
  Ualpha/1 -> Gain18/1, Gain16/1, Mux4/1
  Add5/1 -> Mux4/3
  Gain16/1 -> Add4/2
  Gain18/1 -> Add5/2
  Mux4/1 -> Uabc/1
  Gain15/1 -> Add4/1
  Ubeta/1 -> Gain17/1, Gain15/1
  Gain17/1 -> Add5/1
  Add4/1 -> Mux4/2

== system FluxModel2015a_verify_Q_zhixin/CurrLoop&Observer/Nonlinear Observer/PLL ==
  error : Inport
  Add14 : Sum
  Discrete-Time Integrator2 : DiscreteIntegrator  gainval=1.0/tb  SampleTime=-1  LimitOutput=on  UpperSaturationLimit=PLL_OUTMax_W/Q14  LowerSaturationLimit=-PLL_OUTMax_W/Q14  ICPrevOutput=DiscIntNeverNeededParam  ICPrevScaledInput=DiscIntNeverNeededParam
  Discrete-Time Integrator4 : DiscreteIntegrator  gainval=1.0/tb  SampleTime=-1  UpperSaturationLimit=PLL_OUTMax_W  LowerSaturationLimit=-PLL_OUTMax_W  ICPrevOutput=DiscIntNeverNeededParam  ICPrevScaledInput=DiscIntNeverNeededParam
  Gain : Gain  Gain=PLL_KP
  Gain1 : Gain  Gain=1/Q14
  Gain2 : Gain  Gain=1/Q14
  Gain7 : Gain  Gain=PLL_KI
  Saturation : Saturate  UpperLimit=PLL_OUTMax_W/Q14  LowerLimit=-PLL_OUTMax_W/Q14
  est_theta : Outport
  est_speed : Outport  Port=2
  wires:
  Add14/1 -> Saturation/1
  Saturation/1 -> est_speed/1, Discrete-Time Integrator4/1
  error/1 -> Gain/1, Gain7/1
  Discrete-Time Integrator2/1 -> Add14/2
  Gain/1 -> Gain1/1
  Gain1/1 -> Add14/1
  Gain7/1 -> Gain2/1
  Gain2/1 -> Discrete-Time Integrator2/1
  Discrete-Time Integrator4/1 -> est_theta/1

== system FluxModel2015a_verify_Q_zhixin/CurrLoop&Observer/Nonlinear Observer/PLL1 ==
  error : Inport
  Add14 : Sum
  Discrete-Time Integrator2 : DiscreteIntegrator  gainval=1.0/tb  SampleTime=-1  LimitOutput=on  UpperSaturationLimit=PLL_OUTMax_W  LowerSaturationLimit=-PLL_OUTMax_W  ICPrevOutput=DiscIntNeverNeededParam  ICPrevScaledInput=DiscIntNeverNeededParam
  Discrete-Time Integrator4 : DiscreteIntegrator  gainval=1.0/tb  SampleTime=-1  UpperSaturationLimit=PLL_OUTMax_W  LowerSaturationLimit=-PLL_OUTMax_W  ICPrevOutput=DiscIntNeverNeededParam  ICPrevScaledInput=DiscIntNeverNeededParam
  Gain : Gain  Gain=PLL_KP
  Gain1 : Gain  Gain=1/Q14
  Gain2 : Gain  Gain=1/Q14
  Gain3 : Gain  Gain=10430/Q14
  Gain7 : Gain  Gain=PLL_KI
  Saturation : Saturate  UpperLimit=PLL_OUTMax_W  LowerLimit=-PLL_OUTMax_W
  Scope : Scope
  est_theta : Outport
  est_speed : Outport  Port=2
  wires:
  Discrete-Time Integrator4/1 -> Gain3/1
  Add14/1 -> Saturation/1
  Saturation/1 -> Scope/1, est_speed/1, Discrete-Time Integrator4/1
  error/1 -> Gain/1, Gain7/1
  Discrete-Time Integrator2/1 -> Add14/2
  Gain/1 -> Gain1/1
  Gain1/1 -> Add14/1
  Gain7/1 -> Gain2/1
  Gain2/1 -> Discrete-Time Integrator2/1
  Gain3/1 -> est_theta/1

== system FluxModel2015a_verify_Q_zhixin/CurrLoop&Observer/Nonlinear Observer/clark ==
  Iabc : Inport
  Add : Sum  Inputs=+-
  Demux2 : Demux  Outputs=3
  Gain1 : Gain  Gain=18919
  Gain2 : Gain  Gain=1/Q15
  Ialpha : Outport
  Ibeta : Outport  Port=2
  wires:
  Demux2/3 -> Add/2
  Add/1 -> Gain1/1
  Demux2/1 -> Ialpha/1
  Demux2/2 -> Add/1
  Iabc/1 -> Demux2/1
  Gain1/1 -> Gain2/1
  Gain2/1 -> Ibeta/1

== system FluxModel2015a_verify_Q_zhixin/CurrLoop&Observer/PLLObserver/PLL ==
  error : Inport
  Add14 : Sum
  Discrete-Time Integrator2 : DiscreteIntegrator  gainval=1.0/tb  SampleTime=-1  LimitOutput=on  UpperSaturationLimit=PLL_OUTMax_W  LowerSaturationLimit=-PLL_OUTMax_W  ICPrevOutput=DiscIntNeverNeededParam  ICPrevScaledInput=DiscIntNeverNeededParam
  Discrete-Time Integrator4 : DiscreteIntegrator  gainval=1.0/tb  SampleTime=-1  UpperSaturationLimit=PLL_OUTMax_W  LowerSaturationLimit=-PLL_OUTMax_W  ICPrevOutput=DiscIntNeverNeededParam  ICPrevScaledInput=DiscIntNeverNeededParam
  Gain : Gain  Gain=PLL_KP
  Gain1 : Gain  Gain=1/Q16
  Gain2 : Gain  Gain=1/Q16
  Gain3 : Gain  Gain=10430/Q14
  Gain7 : Gain  Gain=PLL_KI
  Saturation1 : Saturate  UpperLimit=PLL_OUTMax_W  LowerLimit=-PLL_OUTMax_W
  est_theta : Outport
  est_speed : Outport  Port=2
  wires:
  Discrete-Time Integrator4/1 -> Gain3/1
  Add14/1 -> Saturation1/1
  Saturation1/1 -> est_speed/1, Discrete-Time Integrator4/1
  error/1 -> Gain7/1, Gain/1
  Discrete-Time Integrator2/1 -> Add14/2
  Gain/1 -> Gain1/1
  Gain1/1 -> Add14/1
  Gain7/1 -> Gain2/1
  Gain2/1 -> Discrete-Time Integrator2/1
  Gain3/1 -> est_theta/1

== system FluxModel2015a_verify_Q_zhixin/CurrLoop&Observer/PLLObserver/PLL1 ==
  error : Inport
  Add14 : Sum
  Discrete-Time Integrator2 : DiscreteIntegrator  gainval=1.0/tb  SampleTime=-1  LimitOutput=on  UpperSaturationLimit=PLL_OUTMax_W  LowerSaturationLimit=-PLL_OUTMax_W  ICPrevOutput=DiscIntNeverNeededParam  ICPrevScaledInput=DiscIntNeverNeededParam
  Discrete-Time Integrator4 : DiscreteIntegrator  gainval=1.0/tb  SampleTime=-1  UpperSaturationLimit=PLL_OUTMax_W  LowerSaturationLimit=-PLL_OUTMax_W  ICPrevOutput=DiscIntNeverNeededParam  ICPrevScaledInput=DiscIntNeverNeededParam
  Gain : Gain  Gain=PLL_KP
  Gain7 : Gain  Gain=PLL_KI
  Saturation1 : Saturate  UpperLimit=PLL_OUTMax_W  LowerLimit=-PLL_OUTMax_W
  est_theta : Outport
  est_speed : Outport  Port=2
  wires:
  Gain7/1 -> Discrete-Time Integrator2/1
  Discrete-Time Integrator4/1 -> est_theta/1
  Add14/1 -> Saturation1/1
  Saturation1/1 -> est_speed/1, Discrete-Time Integrator4/1
  error/1 -> Gain7/1, Gain/1
  Discrete-Time Integrator2/1 -> Add14/2
  Gain/1 -> Add14/1

== system FluxModel2015a_verify_Q_zhixin/CurrLoop&Observer/ReactivePowerObserver/PLL1 ==
  error : Inport
  Add14 : Sum
  Discrete-Time Integrator2 : DiscreteIntegrator  gainval=1.0/tb  SampleTime=-1  LimitOutput=on  UpperSaturationLimit=PLL_OUTMax_W  LowerSaturationLimit=-PLL_OUTMax_W  ICPrevOutput=DiscIntNeverNeededParam  ICPrevScaledInput=DiscIntNeverNeededParam
  Discrete-Time Integrator4 : DiscreteIntegrator  gainval=1.0/tb  SampleTime=-1  UpperSaturationLimit=PLL_OUTMax_W  LowerSaturationLimit=-PLL_OUTMax_W  ICPrevOutput=DiscIntNeverNeededParam  ICPrevScaledInput=DiscIntNeverNeededParam
  Gain : Gain  Gain=PLL_KP
  Gain7 : Gain  Gain=PLL_KI
  Saturation : Saturate  UpperLimit=PLL_OUTMax_W  LowerLimit=-PLL_OUTMax_W
  est_theta : Outport
  est_speed : Outport  Port=2
  wires:
  Gain7/1 -> Discrete-Time Integrator2/1
  Discrete-Time Integrator4/1 -> est_theta/1
  Add14/1 -> Saturation/1
  Saturation/1 -> est_speed/1, Discrete-Time Integrator4/1
  error/1 -> Gain7/1, Gain/1
  Discrete-Time Integrator2/1 -> Add14/2
  Gain/1 -> Add14/1

== system FluxModel2015a_verify_Q_zhixin/CurrLoop&Observer/SMO/LowPassFilter1 ==
  Input : Inport
  Add : Sum  Inputs=+-
  Add1 : Sum
  Constant : Constant  Value=32767
  Constant1 : Constant  Value=LowPassFilterCoeff_Emf
  Delay6 : Delay  DelayLength=1
  Gain : Gain  Gain=LowPassFilterCoeff_Emf
  Gain3 : Gain  Gain=1/Q15
  Product : Product
  Output : Outport
  wires:
  Delay6/1 -> Gain/1
  Constant/1 -> Add/1
  Constant1/1 -> Add/2
  Input/1 -> Product/1
  Add/1 -> Product/2
  Product/1 -> Add1/1
  Gain/1 -> Add1/2
  Add1/1 -> Gain3/1
  Gain3/1 -> Delay6/1, Output/1

== system FluxModel2015a_verify_Q_zhixin/CurrLoop&Observer/SMO/LowPassFilter2 ==
  Input : Inport
  Add : Sum  Inputs=+-
  Add1 : Sum
  Constant : Constant  Value=32767
  Constant1 : Constant  Value=LowPassFilterCoeff_Emf
  Delay6 : Delay  DelayLength=1
  Gain : Gain  Gain=LowPassFilterCoeff_Emf
  Gain3 : Gain  Gain=1/Q15
  Product : Product
  Output : Outport
  wires:
  Add1/1 -> Gain3/1
  Gain/1 -> Add1/2
  Product/1 -> Add1/1
  Add/1 -> Product/2
  Input/1 -> Product/1
  Constant1/1 -> Add/2
  Constant/1 -> Add/1
  Delay6/1 -> Gain/1
  Gain3/1 -> Output/1, Delay6/1

== system FluxModel2015a_verify_Q_zhixin/CurrLoop&Observer/SMO/PLL2 ==
  error : Inport
  Add14 : Sum
  Discrete-Time Integrator2 : DiscreteIntegrator  gainval=1.0/tb  SampleTime=-1  LimitOutput=on  UpperSaturationLimit=PLL_OUTMax_W  LowerSaturationLimit=-PLL_OUTMax_W  ICPrevOutput=DiscIntNeverNeededParam  ICPrevScaledInput=DiscIntNeverNeededParam
  Discrete-Time Integrator4 : DiscreteIntegrator  gainval=1.0/tb  SampleTime=-1  UpperSaturationLimit=1024  LowerSaturationLimit=0  ICPrevOutput=DiscIntNeverNeededParam  ICPrevScaledInput=DiscIntNeverNeededParam
  Gain : Gain  Gain=PLL_KP
  Gain1 : Gain  Gain=1/Q14
  Gain2 : Gain  Gain=1/Q14
  Gain3 : Gain  Gain=10430/Q14
  Gain7 : Gain  Gain=PLL_KI
  Saturation : Saturate  UpperLimit=PLL_OUTMax_W  LowerLimit=-PLL_OUTMax_W
  Scope : Scope
  est_theta : Outport
  est_speed : Outport  Port=2
  wires:
  Gain/1 -> Gain1/1
  Discrete-Time Integrator2/1 -> Add14/2
  error/1 -> Gain/1, Gain7/1
  Gain7/1 -> Gain2/1
  Gain1/1 -> Add14/1
  Gain2/1 -> Discrete-Time Integrator2/1
  Add14/1 -> Saturation/1
  Discrete-Time Integrator4/1 -> Gain3/1
  Gain3/1 -> est_theta/1
  Saturation/1 -> Scope/1, Discrete-Time Integrator4/1, est_speed/1

== system FluxModel2015a_verify_Q_zhixin/CurrLoop&Observer/SMO/clark1 ==
  Iabc : Inport
  Add : Sum  Inputs=+-
  Demux2 : Demux  Outputs=3
  Gain1 : Gain  Gain=18919
  Gain2 : Gain  Gain=1/Q15
  Ialpha : Outport
  Ibeta : Outport  Port=2
  wires:
  Iabc/1 -> Demux2/1
  Gain2/1 -> Ibeta/1
  Demux2/2 -> Add/1
  Demux2/1 -> Ialpha/1
  Add/1 -> Gain1/1
  Demux2/3 -> Add/2
  Gain1/1 -> Gain2/1

== system FluxModel2015a_verify_Q_zhixin/CurrLoop&Observer/SVCM/clark1 ==
  Iabc : Inport
  Add : Sum  Inputs=+-
  Demux2 : Demux  Outputs=3
  Gain : Gain  Gain=18919
  Gain1 : Gain  Gain=1/Q15
  Ialpha : Outport
  Ibeta : Outport  Port=2
  wires:
  Demux2/3 -> Add/2
  Add/1 -> Gain/1
  Demux2/1 -> Ialpha/1
  Demux2/2 -> Add/1
  Iabc/1 -> Demux2/1
  Gain/1 -> Gain1/1
  Gain1/1 -> Ibeta/1

== system FluxModel2015a_verify_Q_zhixin/CurrLoop&Observer/SVCM/park0 ==
  alpha : Inport
  beta : Inport  Port=2
  theta : Inport  Port=3
  Add : Sum
  Add1 : Sum  Inputs=+-
  Product{,1..3} (4 alike) : Product
  Sin : Trigonometry
  Sin1 : Trigonometry  Operator=cos
  D : Outport
  Q : Outport  Port=2
  wires:
  theta/1 -> Sin1/1, Sin/1
  Product2/1 -> Add1/1
  Sin/1 -> Product3/2, Product1/2
  Add/1 -> D/1
  Product3/1 -> Add1/2
  Sin1/1 -> Product2/2, Product/2
  beta/1 -> Product1/1, Product2/1
  Product1/1 -> Add/2
  Product/1 -> Add/1
  alpha/1 -> Product3/1, Product/1
  Add1/1 -> Q/1
